simulink model "Curva_v4"  (R2019b)
settings: Solver=FixedStepDiscrete  StartTime=0.0  StopTime=35  RelTol=1e-3
model workspace (MAT data in the model file):
  firstWarning = 0
  originalScenarioChecksum = 'FC0F50B9430312EE3AA3C1EBF2A1E89A'
values from neighbouring files (symbols this model uses):
  Cd = 0.33    [initialize.m]
  densidadAire = 1.202    [initialize.m]
  fault_d = 200    [initialize.m]
  frontalArea = 1.873    [initialize.m]
  FV2 = 0    [initialize.m]
  FV3 = 0    [initialize.m]
  Fx0 = 0.015*masa*9.81 + 0.5*densidadAire*frontalArea*Cd*(u0+uw)^2    (= 545.485131)    [initialize.m]
  IV2 = 0    [initialize.m]
  IV3 = 0    [initialize.m]
  masa = 1435    [initialize.m]
  P_ego_init = [4.32 -7.3+1.8]    [initialize.m]
  T2 = 10    [initialize.m]
  T3 = 10    [initialize.m]
  t_gap = 1.5    [initialize.m]
  V_ego_init = 30    [initialize.m]
  Yaw_init = -25    [initialize.m]
undefined symbols (not defined in the file or in its folder): dendriver, DiscIntNeverNeededParam, driving, numdriver, Tsdriver
libraries: simulink_extras x5, drivingscenarioandsensors x3, drivinglib x2, mpcadaslib x1, simulink x1
settings Model: PacingRate=0.750000  Creator=Sun Tzu  LastModifiedBy=Sun Tzu

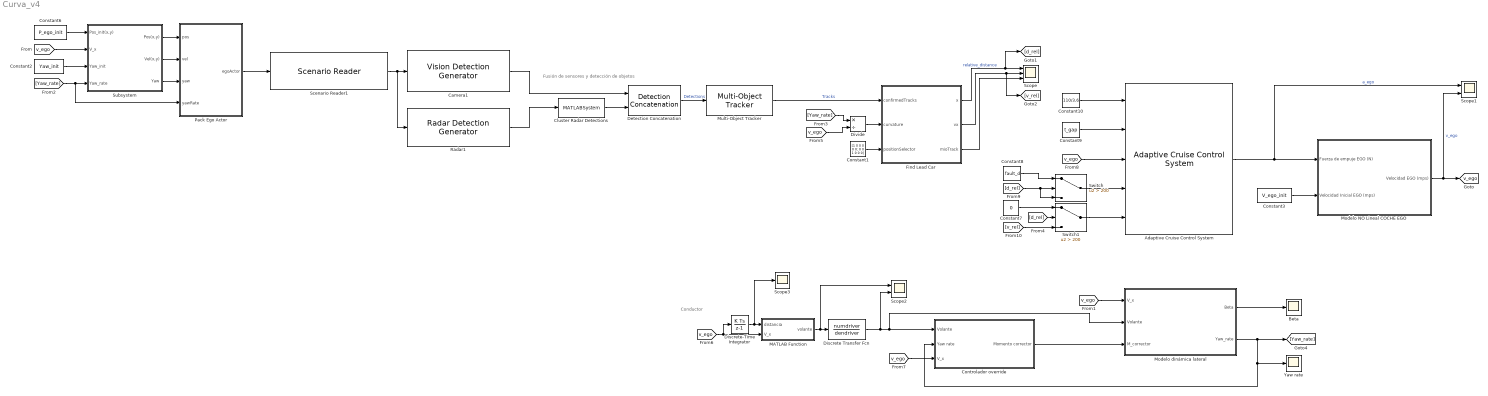
== system Curva_v4 ==
  note: Conductor
  note: Fusión de sensores y detección de objetos
  Adaptive Cruise Control System : mpcadaslib/Adaptive Cruise Control System  EgoModel=tf(0.05,[81.1,1])  InitialEgoVelocity=V_ego_init  DefaultSpacing=10  MaxVelocity=120/3.6  MinAcceleration=Ft_min  amin_ext=off  MaxAcceleration=Ft_max  amax_ext=off  Ts=0.1  PredictionHorizon=30  ControllerBehavior=0.700  suboptimal=off  maxiter=10  datatypeopt=double  optmode=off  trackmode=off
      settings: SourceProductName=Model Predictive Control Toolbox
  Beta : Scope
  Camera1 : drivingscenarioandsensors/Vision Detection Generator  SensorIndex=1  DetectorOutput=Objects only  UpdateInterval=0.05  LaneUpdateInterval=0.1  SensorLocation=[1.9 0]  Height=1.1  Yaw=0  Pitch=1  Roll=0  BusNameSource=Auto  BusName=BusObjectDetections  BusName2Source=Auto  BusName2=BusLaneDetections  MaxNumDetectionsSource=Property  MaxNumDetections=50  MaxNumLanesSource=Property  MaxNumLanes=30  DetectionCoordinates=Ego Cartesian  SimulateUsing=Interpreted execution  MaxRange=100  BoundingBoxAccuracy=5  ProcessNoiseIntensity=5  MaxSpeed=50  MaxAllowedOcclusion=0.5  MinObjectImageSize=[15 15]  DetectionProbability=0.9  FalsePositivesPerImage=0.1  MinLaneImageSize=[20 3]  LaneBoundaryAccuracy=3  HasNoise=on  InitialSeedSource=Repeatable  InitialSeed=0  UsedSeed=0  ActorProfilesSource=MATLAB expression  ActorProfilesParameters=driving.internal.ActorProfilesParameters  ActorProfilesExpression=[struct('ActorID',1,'ClassID',1,'Length',4.7,'Width',1.8,'Height',1.4,'OriginOffset',[-1.35 0 0],'RCSPattern',[10 10;10 10],'RCSAzimuthAngles',[-180 180],'RCSElevationAngles',[-90 90]); struct('ActorID',2,'ClassID',1,'Length',4.7,'Width',1.8,'Height',1.4,'OriginOffset',[-1.35 0 0],'RCSPattern',[10 10;10 10],'RCSAzimuthAngles',[-180 180],'RCSElevationAngles',[-90 90]); struct('ActorID',3,'ClassID',1,'Length',4.7,'Width',1.8,'Height',1.4,'OriginOffset',[-1.35 0 0],'RCSPattern',[10 10;10 10],'RCSAzimuthAngles',[-180 180],'RCSElevationAngles',[-90 90]); struct('ActorID',4,'ClassID',6,'Length',4.7,'Width',1.8,'Height',1.4,'OriginOffset',[-1.35 0 0],'RCSPattern',[10 10;10 10],'RCSAzimuthAngles',[-180 180],'RCSElevationAngles',[-90 90])]  Intrinsics=driving.internal.cameraIntrinsics('FocalLength',[800 799.999999999999],'PrincipalPoint',[320 240],'ImageSize',[480 640],'RadialDistortion',[0 0],'TangentialDistortion',[0 0],'Skew',0)
      settings: SourceProductName=Automated Driving Toolbox
  Cluster Radar Detections : MATLABSystem  System=helperClusterDetections  ClusterSize=5  BusNameSource=Auto  BusName=BusClusterDetections  SimulateUsing=Interpreted execution
      mask Type: helperClusterDetections
      mask Display:
      | disp(['Detection' char(10) 'Clustering']);
      | port_label('input',1,'In');
      | port_label('output',1,'Out');
  Constant1 : Constant  Value=[1 0 0 0 0 0; 0 0 1 0 0 0]
  Constant10 : Constant  Value=110/3.6
  Constant2 : Constant  Value=Yaw_init
  Constant3 : Constant  Value=V_ego_init
  Constant6 : Constant  Value=P_ego_init
  Constant7 : Constant  Value=0
  Constant8 : Constant  Value=fault_d
  Constant9 : Constant  Value=t_gap
  Controlador override : Subsystem
  Detection Concatenation : drivinglib/Detection Concatenation  NumInputs=2  BusNameSource=Auto  BusName=BusDetectionConcatenation1  SimulateUsing=Interpreted execution
      settings: SourceProductName=Automated Driving Toolbox  SourceProductBaseCode=DR
  Discrete Transfer Fcn : DiscreteTransferFcn  Numerator=numdriver  Denominator=dendriver  InitialStates=0.5  SampleTime=Tsdriver
  Discrete-Time Integrator : DiscreteIntegrator  SampleTime=-1  ICPrevOutput=DiscIntNeverNeededParam  ICPrevScaledInput=DiscIntNeverNeededParam
  Divide : Product  Inputs=*/
  Find Lead Car : MATLAB Function  TreatAsAtomicUnit=on
  MATLAB Function : MATLAB Function  TreatAsAtomicUnit=on
  Modelo NO Lineal COCHE EGO : Subsystem
  Modelo dinámica lateral : Subsystem
  Multi-Object Tracker : drivinglib/Multi-Object Tracker  FilterInitializationFcn=helperInitSimulinkDemoFilter  AssignmentThreshold=50  ConfirmationParameters=[ 2, 3 ]  NumCoastingUpdates=5  MaxNumTracks=20  MaxNumSensors=8  TimeInputSource=Auto  HasCostMatrixInput=off  BusNameSource=Auto  BusName=BusMultiObjectTracker1  TentativeTracksOutputPort=off  AllTracksOutputPort=off  SimulateUsing=Interpreted execution
      settings: SourceProductName=Automated Driving Toolbox  SourceProductBaseCode=DR
  Pack Ego Actor : MATLAB Function  TreatAsAtomicUnit=on
  Radar1 : drivingscenarioandsensors/Radar Detection Generator  SensorIndex=2  UpdateInterval=0.05  SensorLocation=[3.7 0]  Height=0.2  Yaw=0  Pitch=0  Roll=0  BusNameSource=Auto  BusName=BusRadarDetectionGenerator  MaxNumDetectionsSource=Property  MaxNumDetections=50  DetectionCoordinates=Ego Cartesian  SimulateUsing=Interpreted execution  AzimuthResolution=4  ElevationResolution=10  RangeResolution=2.5  RangeRateResolution=0.5  AzimuthBiasFraction=0.1  ElevationBiasFraction=0.1  RangeBiasFraction=0.05  RangeRateBiasFraction=0.05  FieldOfView=[15 5]  MaxRange=150  RangeRateLimits=[-100 100]  DetectionProbability=0.9  FalseAlarmRate=1e-06  ReferenceRange=100  ReferenceRCS=0  HasElevation=off  HasRangeRate=on  HasNoise=on  HasFalseAlarms=on  HasOcclusion=on  InitialSeedSource=Repeatable  InitialSeed=0  UsedSeed=0  ActorProfilesSource=MATLAB expression  ActorProfilesParameters=driving.internal.ActorProfilesRadarParameters  ActorProfilesExpression=[struct('ActorID',1,'ClassID',1,'Length',4.7,'Width',1.8,'Height',1.4,'OriginOffset',[-1.35 0 0],'RCSPattern',[10 10;10 10],'RCSAzimuthAngles',[-180 180],'RCSElevationAngles',[-90 90]); struct('ActorID',2,'ClassID',1,'Length',4.7,'Width',1.8,'Height',1.4,'OriginOffset',[-1.35 0 0],'RCSPattern',[10 10;10 10],'RCSAzimuthAngles',[-180 180],'RCSElevationAngles',[-90 90]); struct('ActorID',3,'ClassID',1,'Length',4.7,'Width',1.8,'Height',1.4,'OriginOffset',[-1.35 0 0],'RCSPattern',[10 10;10 10],'RCSAzimuthAngles',[-180 180],'RCSElevationAngles',[-90 90]); struct('ActorID',4,'ClassID',6,'Length',4.7,'Width',1.8,'Height',1.4,'OriginOffset',[-1.35 0 0],'RCSPattern',[10 10;10 10],'RCSAzimuthAngles',[-180 180],'RCSElevationAngles',[-90 90])]
      settings: SourceProductName=Automated Driving Toolbox  SourceProductBaseCode=DR
  Scenario Reader1 : drivingscenarioandsensors/Scenario Reader  ScenarioSource=From file  ScenarioFileName=D:\Sun Tzu\Documents\MIERA\CdV\ControlVehiculosMPC-master\Escenario_Curva\EscenarioCurva_v4.mat  ScenarioVariableName=scenario  OutputCoordinateSystem=Vehicle coordinates  EgoVehicleSource=Input port  EgoVehicleActorID=1  SampleTime=0.05  LaneBoundaryOutput=None  LaneBoundaryDistance=0:0.5:9.5  LaneBoundaryLocation=Center of lane markings  BusNameSource=Auto  BusName=BusActors  BusName2Source=Auto  BusName2=BusLaneBoundaries  SimulateUsing=Interpreted execution
      settings: SourceProductName=Automated Driving Toolbox
  Scope : Scope  NumInputPorts=3
  Scope1 : Scope  NumInputPorts=2
  Scope2 : Scope  NumInputPorts=2
  Scope3 : Scope
  Subsystem : Subsystem
  Switch : Switch  Criteria=u2 > Threshold  Threshold=200
  Switch1 : Switch  Criteria=u2 > Threshold  Threshold=200
  Yaw rate : Scope
  tag scope: v_ego=global
  wires:
  Find Lead Car/1(x) -> [d_rel], Scope/1  "relative_distance"
  Constant10/1 -> Adaptive Cruise Control System/1
  Modelo NO Lineal COCHE EGO/1(Velocidad EGO (mps)) -> Scope1/2, [v_ego]  "v_ego"
  Adaptive Cruise Control System/1 -> Scope1/1, Modelo NO Lineal COCHE EGO/1(Fuerza de empuje EGO (N))  "a_ego"
  Constant1/1 -> Find Lead Car/3(positionSelector)
  [v_ego] -> Adaptive Cruise Control System/3
  Constant3/1 -> Modelo NO Lineal COCHE EGO/2(Velocidad Inicial EGO (mps))
  Switch/1 -> Adaptive Cruise Control System/4
  Constant9/1 -> Adaptive Cruise Control System/2
  [d_rel] -> Switch1/2
  Camera1/1 -> Detection Concatenation/1
  Constant7/1 -> Switch1/1
  [v_rel] -> Switch1/3
  Detection Concatenation/1 -> Multi-Object Tracker/1  "Detections"
  Constant8/1 -> Switch/1
  Find Lead Car/3(mioTrack) -> Scope/3
  Find Lead Car/2(vx) -> [v_rel], Scope/2
  Switch1/1 -> Adaptive Cruise Control System/5
  Radar1/1 -> Cluster Radar Detections/1
  [d_rel] -> Switch/3, Switch/2
  Cluster Radar Detections/1 -> Detection Concatenation/2
  Multi-Object Tracker/1 -> Find Lead Car/1(confirmedTracks)  "Tracks"
  Divide/1 -> Find Lead Car/2(curvature)
  Pack Ego Actor/1(egoActor) -> Scenario Reader1/1
  Discrete Transfer Fcn/1 -> Scope2/2, Modelo dinámica lateral/2(Volante), Controlador override/1(Volante)
  Modelo dinámica lateral/2(Yaw_rate) -> Controlador override/2(Yaw rate), Yaw rate/1, [Yaw_rate]
  Modelo dinámica lateral/1(Beta) -> Beta/1
  [v_ego] -> Modelo dinámica lateral/1(V_x)
  Controlador override/1(Momento corrector) -> Modelo dinámica lateral/3(M_corrector)
  [Yaw_rate] -> Pack Ego Actor/4(yawRate), Subsystem/4(Yaw_rate)
  Constant6/1 -> Subsystem/1(Pos_init(x,y))
  [v_ego] -> Subsystem/2(V_x)
  Constant2/1 -> Subsystem/3(Yaw_init)
  Subsystem/1(Pos(x,y)) -> Pack Ego Actor/1(pos)
  Subsystem/2(Vel(x,y)) -> Pack Ego Actor/2(vel)
  Subsystem/3(Yaw) -> Pack Ego Actor/3(yaw)
  [Yaw_rate] -> Divide/1
  [v_ego] -> Divide/2
  MATLAB Function/1(volante) -> Scope2/1, Discrete Transfer Fcn/1
  [v_ego] -> Discrete-Time Integrator/1, MATLAB Function/2(V_x)
  [v_ego] -> Controlador override/3(V_x)
  Scenario Reader1/1 -> Camera1/1, Radar1/1
  Discrete-Time Integrator/1 -> Scope3/1, MATLAB Function/1(distancia)

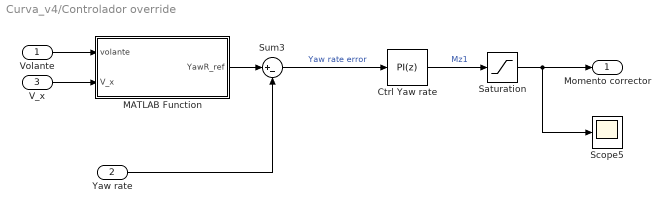
== system Curva_v4/Controlador override ==
  Volante : Inport
  Yaw rate : Inport  Port=2
  V_x : Inport  Port=3
  Ctrl Yaw rate : simulink/Continuous/PID Controller  Controller=PI  Form=Parallel  TimeDomain=Discrete-time  SampleTime=0.01  IntegratorMethod=Forward Euler  FilterMethod=Forward Euler  ControllerParametersSource=internal  P=230124.916945971  I=2828520.69436373  D=0  UseFilter=on  N=100  TunerSelectOption=Transfer Function Based (PID Tuner App)  InitialConditionSource=internal  InitialConditionForIntegrator=0  InitialConditionForFilter=0  DifferentiatorICPrevScaledInput=0  ExternalReset=none  TrackingMode=off  Kt=1  LimitOutput=off  UpperSaturationLimit=inf  LowerSaturationLimit=-inf  LinearizeAsGain=on  AntiWindupMode=none  Kb=1  POutMin=[]  POutMax=[]  IOutMin=[]  IOutMax=[]  DOutMin=[]  DOutMax=[]  NOutMin=[]  NOutMax=[]  SumOutMin=[]  SumOutMax=[]  SaturationOutMin=[]  SaturationOutMax=[]  PParamMin=[]  PParamMax=[]  IParamMin=[]  IParamMax=[]  DParamMin=[]  DParamMax=[]  NParamMin=[]  NParamMax=[]  KbParamMin=[]  KbParamMax=[]  KtParamMin=[]  KtParamMax=[]  KbOutMin=[]  KbOutMax=[]  KtOutMin=[]  KtOutMax=[]  IntegratorOutMin=[]  IntegratorOutMax=[]  FilterOutMin=[]  FilterOutMax=[]  SumI1OutMin=[]  SumI1OutMax=[]  SumI2OutMin=[]  SumI2OutMax=[]  SumI3OutMin=[]  SumI3OutMax=[]  SumI4OutMin=[]  SumI4OutMax=[]  SumDOutMin=[]  SumDOutMax=[]  DifferentiatorOutMin=[]  DifferentiatorOutMax=[]  FilterDiffOutCoefMin=[]  FilterDiffOutCoefMax=[]  ReciprocalOutMin=[]  ReciprocalOutMax=[]  SumDenOutMin=[]  SumDenOutMax=[]  SumNumOutMin=[]  SumNumOutMax=[]  DivideOutMin=[]  DivideOutMax=[]  IntegratorContinuousStateAttributes=''  IntegratorStateMustResolveToSignalObject=off  IntegratorRTWStateStorageClass=Auto  FilterContinuousStateAttributes=''  FilterStateMustResolveToSignalObject=off  FilterRTWStateStorageClass=Auto  ParallelPVariant=InternalParameters  IdealPVariant=Disabled  IVariant=InternalParameters  DVariant=Disabled  IntegratorVariant=Discrete  SatVariant=Disabled  AWVariant=Passthrough  PCopyVariant=Disabled  TRVariant=Disabled  FdbkBlocksVariant=Forward  IdealPFdbkVariant=Disabled  SatFdbkVariant=Disabled  DerivativeFilterVariant=Disabled  NVariant=Disabled  NCopyVariant=Disabled_SignalSpec  FilterICVariant=Disabled  IntegratorICVariant=InternalICs  ExternalResetVariant=Disabled  TRSumVariant=Passthrough  SumFdbkVariant=Disabled  SumVariant=Sum_PI
  MATLAB Function : MATLAB Function  TreatAsAtomicUnit=on
  Saturation : Saturate  UpperLimit=5000  LowerLimit=-5000
  Scope5 : Scope
  Sum3 : Sum  Inputs=|+-
  Momento corrector : Outport
  wires:
  Saturation/1 -> Momento corrector/1, Scope5/1
  Sum3/1 -> Ctrl Yaw rate/1  "Yaw rate error"
  Ctrl Yaw rate/1 -> Saturation/1  "Mz1"
  MATLAB Function/1(YawR_ref) -> Sum3/1
  Volante/1 -> MATLAB Function/1(volante)
  Yaw rate/1 -> Sum3/2
  V_x/1 -> MATLAB Function/2(V_x)

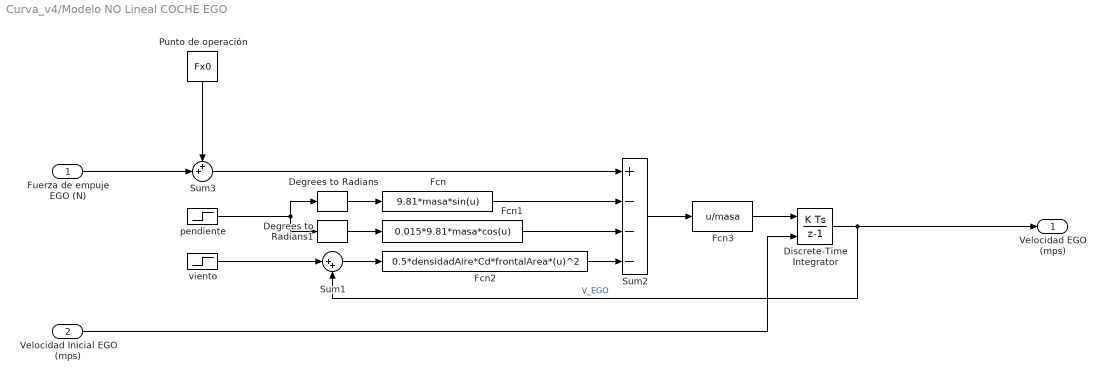
== system Curva_v4/Modelo NO Lineal COCHE EGO ==
  Fuerza de empuje EGO (N) : Inport
  Velocidad Inicial EGO (mps) : Inport  Port=2
  Degrees to Radians : simulink_extras/Transformations/Degrees to Radians
  Degrees to Radians1 : simulink_extras/Transformations/Degrees to Radians
  Discrete-Time Integrator : DiscreteIntegrator  InitialConditionSource=external  SampleTime=-1  ICPrevOutput=DiscIntNeverNeededParam  ICPrevScaledInput=DiscIntNeverNeededParam
  Fcn : Fcn  Expr=9.81*masa*sin(u)
  Fcn1 : Fcn  Expr=0.015*9.81*masa*cos(u)
  Fcn2 : Fcn  Expr=0.5*densidadAire*Cd*frontalArea*(u)^2
  Fcn3 : Fcn  Expr=u/masa
  Punto de operación : Constant  Value=Fx0
  Sum1 : Sum  Inputs=|++
  Sum2 : Sum  Inputs=+---
  Sum3 : Sum  Inputs=++|
  pendiente : Step  Time=T2  Before=IV2  After=FV2  SampleTime=0
  viento : Step  Time=T3  Before=IV3  After=FV3  SampleTime=0
  Velocidad EGO (mps) : Outport  VectorParamsAs1DForOutWhenUnconnected=off
  wires:
  Discrete-Time Integrator/1 -> Velocidad EGO (mps)/1, Sum1/2  "V_EGO"
  Velocidad Inicial EGO (mps)/1 -> Discrete-Time Integrator/2
  Punto de operación/1 -> Sum3/1
  Fuerza de empuje EGO (N)/1 -> Sum3/2
  Sum3/1 -> Sum2/1
  viento/1 -> Sum1/1
  Sum1/1 -> Fcn2/1
  Fcn1/1 -> Sum2/3
  Degrees to Radians1/1 -> Fcn1/1
  Fcn3/1 -> Discrete-Time Integrator/1
  Fcn/1 -> Sum2/2
  pendiente/1 -> Degrees to Radians/1, Degrees to Radians1/1
  Degrees to Radians/1 -> Fcn/1
  Sum2/1 -> Fcn3/1
  Fcn2/1 -> Sum2/4

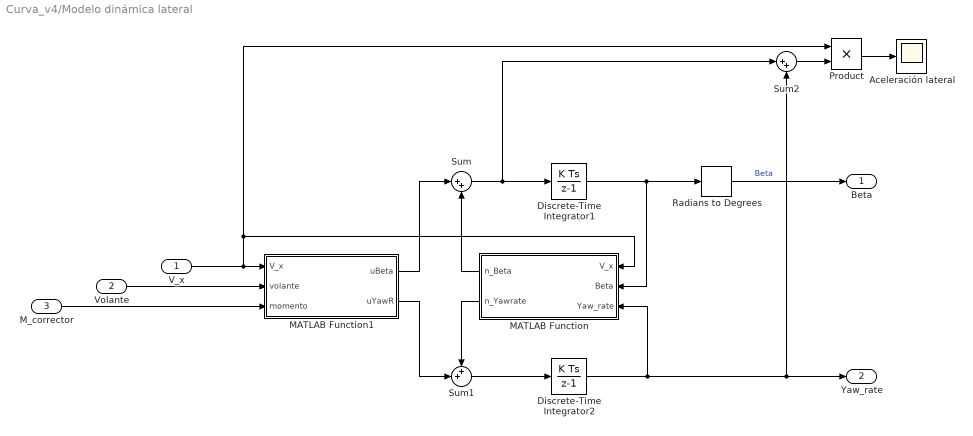
== system Curva_v4/Modelo dinámica lateral ==
  V_x : Inport
  Volante : Inport  Port=2
  M_corrector : Inport  Port=3
  Aceleración lateral : Scope
  Discrete-Time Integrator1 : DiscreteIntegrator  InitialCondition=-0.011341149479459  SampleTime=0.01  ICPrevOutput=DiscIntNeverNeededParam  ICPrevScaledInput=DiscIntNeverNeededParam
  Discrete-Time Integrator2 : DiscreteIntegrator  InitialCondition=0.08679  SampleTime=0.01  ICPrevOutput=DiscIntNeverNeededParam  ICPrevScaledInput=DiscIntNeverNeededParam
  MATLAB Function : MATLAB Function  TreatAsAtomicUnit=on
  MATLAB Function1 : MATLAB Function  TreatAsAtomicUnit=on
  Product : Product
  Radians to Degrees : simulink_extras/Transformations/Radians to Degrees
  Sum : Sum  Inputs=|++
  Sum1 : Sum  Inputs=++|
  Sum2 : Sum  Inputs=|++
  Beta : Outport
  Yaw_rate : Outport  Port=2
  wires:
  Discrete-Time Integrator2/1 -> MATLAB Function/3(Yaw_rate), Yaw_rate/1, Sum2/2
  Sum2/1 -> Product/2
  V_x/1 -> Product/1, MATLAB Function/1(V_x), MATLAB Function1/1(V_x)
  MATLAB Function/1(n_Beta) -> Sum/2
  Product/1 -> Aceleración lateral/1
  MATLAB Function/2(n_Yawrate) -> Sum1/1
  MATLAB Function1/1(uBeta) -> Sum/1
  Discrete-Time Integrator1/1 -> MATLAB Function/2(Beta), Radians to Degrees/1
  MATLAB Function1/2(uYawR) -> Sum1/2
  Sum1/1 -> Discrete-Time Integrator2/1
  Sum/1 -> Discrete-Time Integrator1/1, Sum2/1
  M_corrector/1 -> MATLAB Function1/3(momento)
  Volante/1 -> MATLAB Function1/2(volante)
  Radians to Degrees/1 -> Beta/1  "Beta"

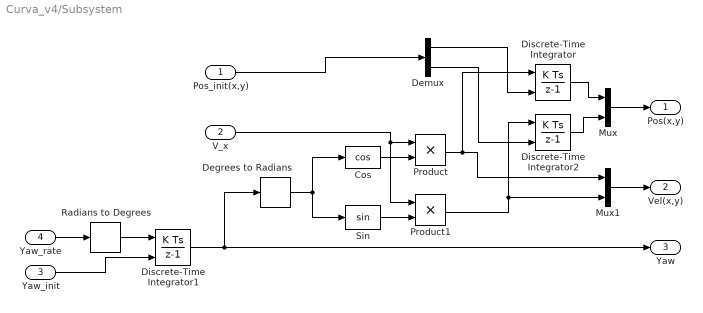
== system Curva_v4/Subsystem ==
  Pos_init(x,y) : Inport
  V_x : Inport  Port=2
  Yaw_init : Inport  Port=3
  Yaw_rate : Inport  Port=4
  Cos : Trigonometry  Operator=cos
  Degrees to Radians : simulink_extras/Transformations/Degrees to Radians
  Demux : Demux  Outputs=2
  Discrete-Time Integrator : DiscreteIntegrator  InitialConditionSource=external  InitialCondition=5  SampleTime=-1  ICPrevOutput=DiscIntNeverNeededParam  ICPrevScaledInput=DiscIntNeverNeededParam
  Discrete-Time Integrator1 : DiscreteIntegrator  InitialConditionSource=external  SampleTime=-1  ICPrevOutput=DiscIntNeverNeededParam  ICPrevScaledInput=DiscIntNeverNeededParam
  Discrete-Time Integrator2 : DiscreteIntegrator  InitialConditionSource=external  SampleTime=-1  ICPrevOutput=DiscIntNeverNeededParam  ICPrevScaledInput=DiscIntNeverNeededParam
  Mux : Mux  Inputs=2
  Mux1 : Mux  Inputs=2
  Product : Product
  Product1 : Product
  Radians to Degrees : simulink_extras/Transformations/Radians to Degrees
  Sin : Trigonometry
  Pos(x,y) : Outport
  Vel(x,y) : Outport  Port=2
  Yaw : Outport  Port=3
  wires:
  Product/1 -> Discrete-Time Integrator/1, Mux1/1
  Discrete-Time Integrator1/1 -> Yaw/1, Degrees to Radians/1
  Discrete-Time Integrator/1 -> Mux/1
  Product1/1 -> Discrete-Time Integrator2/1, Mux1/2
  Demux/2 -> Discrete-Time Integrator2/2
  V_x/1 -> Product1/1, Product/1
  Yaw_rate/1 -> Radians to Degrees/1
  Discrete-Time Integrator2/1 -> Mux/2
  Demux/1 -> Discrete-Time Integrator/2
  Cos/1 -> Product/2
  Sin/1 -> Product1/2
  Pos_init(x,y)/1 -> Demux/1
  Yaw_init/1 -> Discrete-Time Integrator1/2
  Mux1/1 -> Vel(x,y)/1
  Mux/1 -> Pos(x,y)/1
  Radians to Degrees/1 -> Discrete-Time Integrator1/1
  Degrees to Radians/1 -> Cos/1, Sin/1

== matlab function Curva_v4/Find Lead Car ==
  data: confirmedTracks input; x output double size=[1 1]; vx output size=[1 1]; curvature input; mioTrack output; positionSelector input
function [x,vx,mioTrack] = findLeadCar(confirmedTracks, curvature, positionSelector)
% This function finds the lead car: a car in front of the ego car that
% satisfies all the criteria below:
% * Within the ego car's lane.
% * In front of the ego car.
% * Closest to the ego car.

% Important notes:
% 1. If you change state definition, change the following:
%       State = [x;vx;y;vy;z;vz] (3D constant velocity)
numStates = 6;

% 2. The lane is defined using a parabolic model, where y=ax^2+bx+c. a is
%    equal to half the road curvature, b=0, and c is the offset of the lane
%    boundaries relative to the ego car. Overall lane width is assumed to
%    be 3.6m, typical highway lane width.
laneWidth = 3.6;

% 3. The ego car is assumed to be traveling in the middle of its lane, with
%    1.8m on each side of it. So, c=+1.8m for the left lane boundary and
%    -1.8m for the right lane boundary.
halfLaneWidth = laneWidth/2;

% Initialize outputs and parameters
maxX = cast(1000, 'like', confirmedTracks.Tracks(1).State);  % Far enough forward so that no track is expected to exceed this distance
trackID = 0;

for i = 1:confirmedTracks.NumTracks
    position = positionSelector * confirmedTracks.Tracks(i).State;
    x = position(1); % Longitudinal position of the track relative to ego
    y = position(2); % Lateral position of the track relative to ego
    
    if x < maxX && x > 0 % No point checking otherwise
        yleftLane  = polyval([curvature/2, 0,  halfLaneWidth],x); % Half a lane to the left
        yrightLane = polyval([curvature/2, 0, -halfLaneWidth],x); % Half a lane to the right
        
        % Find a new lead car
        if (yrightLane <= y) && (y <= yleftLane)
            maxX = x;
            trackID = i;
        end
    end
end

if trackID>0
    mioState = confirmedTracks.Tracks(trackID).State;
else
    mioState = inf(numStates,1,'like',confirmedTracks.Tracks(1).State);
end

% Output:
x = mioState(1);    % Longitudinal position of the lead car
vx = mioState(2);   % Longitudinal velocity of the lead car
mioTrack = trackID; % Index of the most important track

== matlab function Curva_v4/Modelo dinámica lateral/MATLAB Function ==
  data: V_x input; n_Beta output; Beta input; n_Yawrate output; Yaw_rate input
function [n_Beta, n_Yawrate] = matrizA(V_x,Beta,Yaw_rate)

masa = 1435;
L = 2.54;
a = 1.14;
b = L - a;
I_z = 2420;
C_af = 44000;
C_ar = 47000;

A = [-2*(C_af+C_ar)/(masa*V_x) 2*(-a*C_af + b*C_ar)/(masa*V_x^2)-1; ...
    2*(-a*C_af + b*C_ar)/I_z -2*(a^2*C_af + b^2*C_ar)/(I_z*V_x)];

n_estados = A*[Beta; Yaw_rate];
n_Beta = n_estados(1);
n_Yawrate = n_estados(2);

== matlab function Curva_v4/Modelo dinámica lateral/MATLAB Function1 ==
  data: V_x input; uBeta output; volante input; momento input; uYawR output
function [uBeta, uYawR] = matrizB(V_x,volante,momento)

masa = 1435;
a = 1.14;
I_z = 2420;
C_af = 44000;
C_ar = 47000;

B = [2*C_af/(masa*V_x) 0; 2*a*C_ar/I_z 1/I_z];

us = B*[volante; momento];
uBeta = us(1);
uYawR = us(2);

== matlab function Curva_v4/Controlador override/MATLAB Function ==
  data: volante input; YawR_ref output; V_x input
function YawR_ref = YawR_ref(volante,V_x)

masa = 1435;
L = 2.54;
a = 1.14;
b = L - a;
C_af = 44000;
C_ar = 47000;

YawR_ref = V_x/(L+masa/L*(b/C_af-a/C_ar)*V_x^2)*volante;

== matlab function Curva_v4/Pack Ego Actor ==
  data: pos input; egoActor output Bus: BusActors1Actors size=1; vel input; yaw input; yawRate input
function egoActor = packEgo(pos,vel,yaw,yawRate)
% Pack ego information into a single ego actor bus
%
% Imoprtant note:
% Output is a bus of type BusActorsActors. This is the same bus used by the
% Scenario Reader to output an individual actor. If you change the
% output bus name of Scenario Reader, change the output bus name here
% as well by clicking on 'Edit Data' in the menu above.

egoActor = struct(...
    'ActorID',1,...
    'Position', [pos(1) pos(2) 0], ...
    'Velocity', [vel(1) vel(2) 0], ...
    'Roll', 0, ...
    'Pitch', 0, ...
    'Yaw', yaw, ...
    'AngularVelocity', [0 0 yawRate]);

== matlab function Curva_v4/MATLAB Function ==
  data: distancia input; volante output; V_x input
function volante = conductor(distancia,V_x)

masa = 1435;
L = 2.54;
a = 1.14;
b = L - a;
C_af = 44000;
C_ar = 47000;

if distancia < 411+15
    R = 351.8;
    volante = (L+masa/L*(b/C_af-a/C_ar)*V_x^2)/R;
elseif distancia < 411+15+170
    volante = 0;
elseif distancia < 840
    R = -188+3.6;
    volante = (L+masa/L*(b/C_af-a/C_ar)*V_x^2)/R;
else
    R = -188-3.6;
    volante = (L+masa/L*(b/C_af-a/C_ar)*V_x^2)/R;
end
